simulink subsystem "ROT"  (R2021a)
settings: Solver=VariableStepAuto  StartTime=0.0  StopTime=10.0  RelTol=1e-3
libraries: hdlBasic x27
settings Model: Creator=ckk5  LastModifiedBy=ckk5

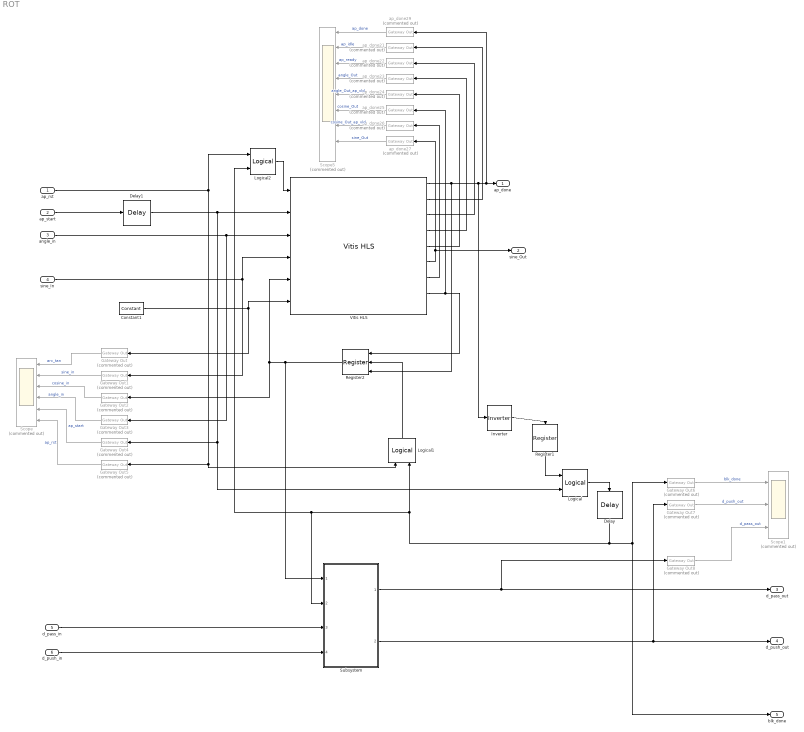
== system ROT ==
  ap_rst : Inport
  ap_start : Inport  Port=2
  angle_in : Inport  Port=3
  sine_In : Inport  Port=4
  d_pass_in : Inport  Port=5
  d_push_in : Inport  Port=6
  Constant1 : hdlBasic/Constant  const=0  gui_display_data_type=Boolean  arith_type=Boolean  n_bits=16  bin_pt=14  preci_type=Single  exp_width=8  frac_width=24  explicit_period=off  period=1  XmcBlockStatus=1  maskContainerNames=tabcontainer1  block_type=constant  block_config=sysgen:Constant_config
  Delay : hdlBasic/Delay  rst=off  en=off  latency=1  reg_retiming=off  XmcBlockStatus=1  maskContainerNames=group1  block_type=delay  block_config=sysgen:Delay_config
  Delay1 : hdlBasic/Delay  rst=off  en=off  latency=1  reg_retiming=off  XmcBlockStatus=1  maskContainerNames=group1  block_type=delay  block_config=sysgen:Delay_config
  Gateway Out{,1..8} (9 alike) : hdlBasic/Gateway Out  Commented=on  inherit_from_input=off  hdl_port=on  rows=1  columns=1  UseAsDAC=off  DACChannel='1'  interface=None  automatic_assignment=on  address_offset=hex2dec('00')  intf_name=''  intf_description=''  timing_constraint=None  locs_specified=off  LOCs={}  io_standard={}  XmcBlockStatus=1  maskContainerNames=group4  block_type=gatewayout  block_config=sysgen:gateway_out_config  block_width_w=590  block_height_w=620  block_width=620  block_height=750
  Inverter : hdlBasic/Inverter  en=off  latency=0  XmcBlockStatus=1  maskContainerNames=group2  block_type=inv  block_config=sysgen:Inverter_config
  Logical : hdlBasic/Logical  logical_function=NOR  inputs=2  en=off  latency=0  precision=Full  arith_type=Unsigned  n_bits=16  bin_pt=0  align_bp=on  overflow=[]  quantization=[]  XmcBlockStatus=1  maskContainerNames=tabcontainer1  block_type=logical  block_config=sysgen:Logical_config
  Logical1 : hdlBasic/Logical  logical_function=OR  inputs=2  en=off  latency=0  precision=Full  arith_type=Unsigned  n_bits=16  bin_pt=0  align_bp=on  overflow=[]  quantization=[]  XmcBlockStatus=1  maskContainerNames=tabcontainer1  block_type=logical  block_config=sysgen:Logical_config
  Logical2 : hdlBasic/Logical  logical_function=OR  inputs=2  en=off  latency=0  precision=Full  arith_type=Unsigned  n_bits=16  bin_pt=0  align_bp=on  overflow=[]  quantization=[]  XmcBlockStatus=1  maskContainerNames=tabcontainer1  block_type=logical  block_config=sysgen:Logical_config
  Register1 : hdlBasic/Register  init=1  rst=off  en=off  XmcBlockStatus=1  maskContainerNames=tabcontainer1  block_type=register  block_config=sysgen:Register_config
  Register2 : hdlBasic/Register  init=0  rst=on  en=on  XmcBlockStatus=1  maskContainerNames=tabcontainer1  block_type=register  block_config=sysgen:Register_config
  Scope : Scope  Commented=on  NumInputPorts=6
  Scope1 : Scope  Commented=on  NumInputPorts=3
  Scope5 : Scope  Commented=on  NumInputPorts=9
  Subsystem : Subsystem  ReferencedSubsystem=Output_Selector_Simple
  Vitis HLS : hdlBasic/Vitis HLS  anytable='C:\ELEC522\Cameron\lab_five\vitis_hls\lab_five\solution1'  fast_sim=off  display_datatype=on  rate_propagation_method=Simulink system period  model_file_path=''  latency=1  block_type=vitis_hls
      settings: infoedit=This block allows including C,C++ and SystemC source files in System Generator for DSP designs.
  ap_done{21..27,29} (8 alike) : hdlBasic/Gateway Out  Commented=on  inherit_from_input=off  hdl_port=on  rows=1  columns=1  UseAsDAC=off  DACChannel='1'  interface=None  automatic_assignment=on  address_offset=hex2dec('00')  intf_name=''  intf_description=''  timing_constraint=None  locs_specified=off  LOCs={}  io_standard={}  XmcBlockStatus=1  maskContainerNames=group4  block_type=gatewayout  block_config=sysgen:gateway_out_config  block_width_w=590  block_height_w=620  block_width=620  block_height=750
  ap_done : Outport
  sine_Out : Outport  Port=2
  d_pass_out : Outport  Port=3
  d_push_out : Outport  Port=4
  blk_done : Outport  Port=5
  wires:
  Vitis HLS/7 -> ap_done26/1
  Vitis HLS/5 -> ap_done24/1
  Vitis HLS/1 -> Inverter/1, ap_done/1, ap_done29/1, Register2/3
  Vitis HLS/2 -> ap_done21/1
  Vitis HLS/3 -> ap_done22/1
  Vitis HLS/6 -> ap_done27/1, sine_Out/1
  Vitis HLS/4 -> ap_done23/1
  Constant1/1 -> Gateway Out/1, Vitis HLS/6
  Vitis HLS/8 -> ap_done25/1, Register2/1
  ap_rst/1 -> Gateway Out5/1, Logical1/1, Logical2/1
  angle_in/1 -> Vitis HLS/3, Gateway Out3/1
  Gateway Out/1 -> Scope/1  "arc_tan"
  Gateway Out1/1 -> Scope/2  "sine_in"
  Gateway Out2/1 -> Scope/3  "cosine_in"
  Register2/1 -> Vitis HLS/5, Gateway Out2/1, Subsystem/1
  Gateway Out3/1 -> Scope/4  "angle_in"
  Gateway Out4/1 -> Scope/5  "ap_start"
  Gateway Out5/1 -> Scope/6  "ap_rst"
  ap_done22/1 -> Scope5/3  "ap_ready"
  ap_done24/1 -> Scope5/5  "angle_Out_ap_vld"
  ap_done25/1 -> Scope5/6  "cosine_Out"
  ap_done29/1 -> Scope5/1  "ap_done"
  ap_done21/1 -> Scope5/2  "ap_idle"
  ap_done27/1 -> Scope5/8  "sine_Out"
  ap_done26/1 -> Scope5/7  "cosine_Out_ap_vld"
  ap_done23/1 -> Scope5/4  "angle_Out"
  Inverter/1 -> Register1/1
  Logical1/1 -> Register2/2
  Gateway Out8/1 -> Scope1/3  "d_pass_out"
  Gateway Out7/1 -> Scope1/2  "d_push_out"
  Gateway Out6/1 -> Scope1/1  "blk_done"
  d_pass_in/1 -> Subsystem/3
  d_push_in/1 -> Subsystem/4
  Subsystem/1 -> d_pass_out/1, Gateway Out8/1
  Subsystem/2 -> Gateway Out7/1, d_push_out/1
  Logical2/1 -> Vitis HLS/1
  Logical/1 -> Delay/1
  Delay/1 -> Logical1/2, Logical2/2, Subsystem/2, blk_done/1, Gateway Out6/1
  sine_In/1 -> Gateway Out1/1, Vitis HLS/4
  ap_start/1 -> Delay1/1
  Register1/1 -> Logical/1
  Delay1/1 -> Vitis HLS/2, Gateway Out4/1, Logical/2
